simulink model "PID_Controller"  (R2020b)
settings: Solver=FixedStepAuto  StartTime=0.0  StopTime=10.0  FixedStep=0.001  RelTol=1e-3
settings Model: Creator=shivanshu shukla  LastModifiedBy=shivanshu shukla
settings DataIOCC: SaveOutput=off  SaveTime=off

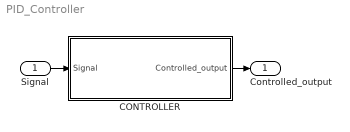
== system PID_Controller ==
  Signal : Inport  OutDataTypeStr=double  PortDimensions=1
  CONTROLLER : Subsystem
  Controlled_output : Outport  OutDataTypeStr=double  PortDimensions=1  SampleTime=[0.001,0]
  wires:
  Signal/1 -> CONTROLLER/1(Signal)
  CONTROLLER/1(Controlled_output) -> Controlled_output/1

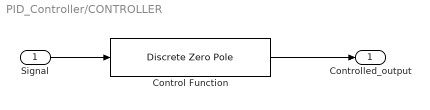
== system PID_Controller/CONTROLLER ==
  Signal : Inport  OutDataTypeStr=double  PortDimensions=1  SampleTime=[0,1]
  Control Function : DiscreteZeroPole  Zeros=[0.95 0.8 0.8]  Poles=[-0.98 0.6 1]  Gain=800  SampleTime=0.001
  Controlled_output : Outport  OutDataTypeStr=double  PortDimensions=1  SampleTime=[0.001,0]
  wires:
  Control Function/1 -> Controlled_output/1
  Signal/1 -> Control Function/1
